simulink model "simulink_model"  (R2022b)
settings: Solver=VariableStepAuto  StartTime=0.0  StopTime=5*N  RelTol=1e-3
libraries: cstblocks x1
settings Model: Creator=chuan  LastModifiedBy=chuan

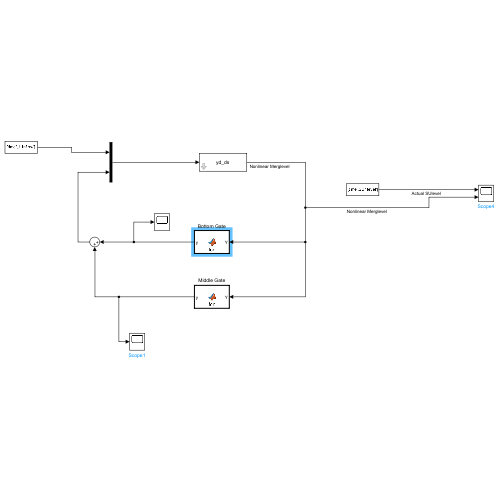
[thumbnail: Simulink's stored preview of the top-level diagram]
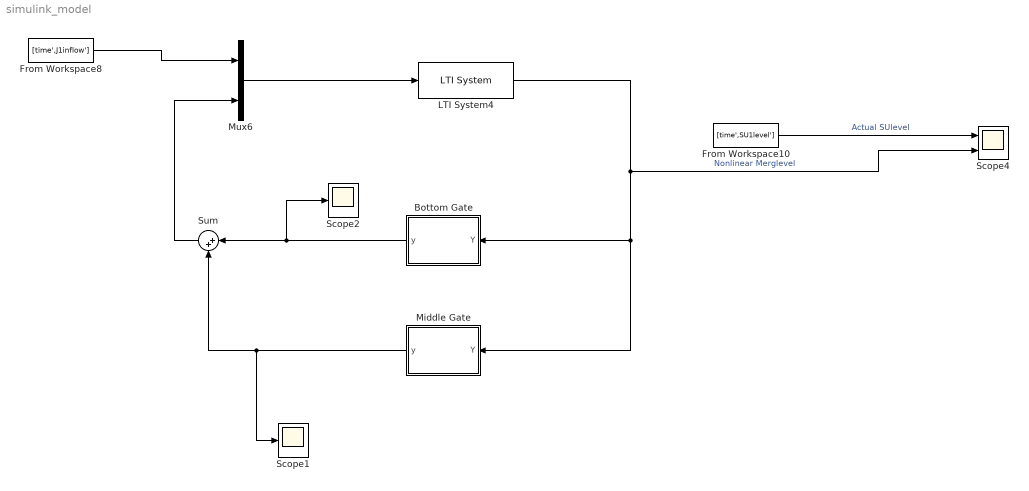
== system simulink_model ==
  Bottom Gate : MATLAB Function  TreatAsAtomicUnit=on
  From Workspace10 : FromWorkspace  VariableName=[time',SU1level']
  From Workspace8 : FromWorkspace  VariableName=[time',J1inflow']
  LTI System4 : cstblocks/LTI System  sys=yd_ds  IC=[]
  Middle Gate : MATLAB Function  TreatAsAtomicUnit=on
  Mux6 : Mux  Inputs=2
  Scope1 : Scope
  Scope2 : Scope
  Scope4 : Scope  NumInputPorts=2
  Sum : Sum  Inputs=|++
  wires:
  From Workspace8/1 -> Mux6/1
  From Workspace10/1 -> Scope4/1  "Actual SUlevel"
  Mux6/1 -> LTI System4/1
  LTI System4/1 -> Middle Gate/1(Y), Bottom Gate/1(Y), Scope4/2  "Nonlinear Merglevel"
  Bottom Gate/1(y) -> Scope2/1, Sum/1
  Middle Gate/1(y) -> Scope1/1, Sum/2
  Sum/1 -> Mux6/2

== matlab function simulink_model/Bottom Gate ==
  data: Y input; y output
function y = fcn(Y)
Cd = 0.65;
A0 = 1;
g = 9.81;
Z0 = 0;
Yfull = 1;
H_star = Z0 + Yfull;

Y = max(Y,0);
H1 = Y + Z0;

if H1 >= H_star
    He = H1 - (Z0 + Yfull/2);
    y = Cd*A0*sqrt(2*g*He);
else
    CwL = (Cd*A0*sqrt(g))/(Yfull);
    y = CwL*(H1-Z0)^(1.5);
end

== matlab function simulink_model/Middle Gate ==
  data: Y input; y output
function y = fcn(Y)
Cd = 0.65;
A0 = 25;
g = 9.81;
Z0 = 0;
Yfull = 5;
H_star = Z0 + Yfull;

Y = max(Y,0);
H1 = Y + Z0;

% if H1 >= H_star + 10
%     He = H1 - (Z0 + Yfull/2);
%     y = Cd*A0*sqrt(2*g*He);
% elseif H1 > 10 && H1 < 15
%     CwL = (Cd*A0*sqrt(g))/(Yfull);
%     y = CwL*(H1-Z0)^(1.5);
% else 
%     y = 0;
% end

if H1 >= H_star
    He = H1 - (Z0 + Yfull/2);
    y = Cd*A0*sqrt(2*g*He);
else
    CwL = (Cd*A0*sqrt(g))/(Yfull);
    y = CwL*(H1-Z0)^(1.5);
end
